simulink model "manifold"  (Simulink 8.3)
settings: Solver=ode45  StartTime=0.0  StopTime=100  FixedStep=0.001  MaxStep=1  RelTol=1e-3
values from neighbouring files (symbols this model uses):
  Cp = 1003    [InitPar.m]
  Cv = 717    [InitPar.m]
  epsilon = 10    [InitPar.m]
  kappa = Cp/Cv    (= 1.39888423989)    [InitPar.m]
  Pe = 8.36 * 10^4    (= 83600)    [InitPar.m]
  R = 287    [InitPar.m]
  theta_e = 400    [InitPar.m]
  theta_in = 295    [InitPar.m]
  Vdot_ideal = 0.024546    [InitPar.m]    (also in manifold_optimisation.m = X(2); simulation_error.m = simulation_parameters(2))
  Vm = 0.0063815    [InitPar.m]    (also in manifold_optimisation.m = X(1); simulation_error.m = simulation_parameters(1))
settings Model: Creator=daniel  LastModifiedBy=daniel
settings DataIOCC: SignalLoggingSaveFormat=Dataset
settings DebuggingCC: UnderspecifiedInitializationDetection=Simplified  StateNameClashWarn=none
settings GRTTargetCC: CombineOutputUpdateFcns=on  GRTInterface=off
settings ConfigurationSet: Description=SimMechanics 2G

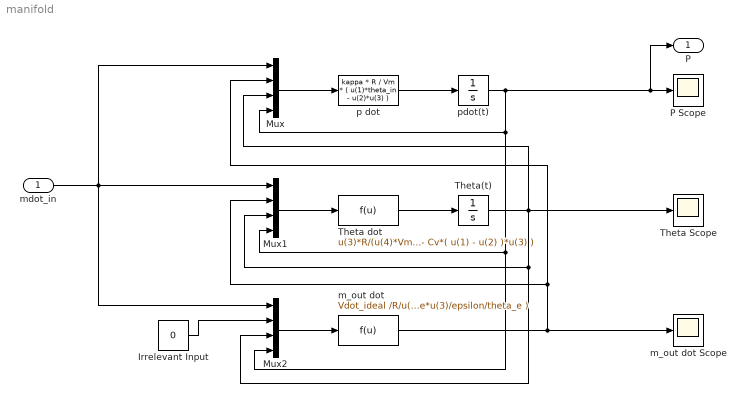
== system manifold ==
  mdot_in : Inport
  Irrelevant Input : Constant  Value=0
  Mux : Mux
  Mux1 : Mux
  Mux2 : Mux
  P Scope : Scope
      settings: YMin=2.5e+08  YMax=1.1e+09
  Theta Scope : Scope
  Theta dot : Fcn  Expr=u(3)*R/(u(4)*Vm*Cv) * ( Cp*u(1)*theta_in - Cp*u(2)*u(3) - Cv*( u(1) - u(2) )*u(3) )
  Theta(t) : Integrator  InitialCondition=theta_in
  m_out dot : Fcn  Expr=Vdot_ideal /R/u(3) * ( u(4)*(epsilon+1)/epsilon - Pe*u(3)/epsilon/theta_e )
  m_out dot Scope : Scope
      settings: TimeRange=0.3499999999999996  YMin=0  YMax=0.003  SaveName=ScopeData2
  p dot : Fcn  Expr=kappa * R / Vm * ( u(1)*theta_in - u(2)*u(3) )
  pdot(t) : Integrator  InitialCondition=Pe
  P : Outport
  wires:
  Mux1/1 -> Theta dot/1
  Mux2/1 -> m_out dot/1
  Mux/1 -> p dot/1
  p dot/1 -> pdot(t)/1
  Theta dot/1 -> Theta(t)/1
  pdot(t)/1 -> Mux/4, Mux1/4, Mux2/4, P/1, P Scope/1
  Theta(t)/1 -> Mux/3, Theta Scope/1, Mux1/3, Mux2/3
  m_out dot/1 -> m_out dot Scope/1, Mux/2, Mux1/2
  mdot_in/1 -> Mux2/1, Mux/1, Mux1/1
  Irrelevant Input/1 -> Mux2/2
